simulink model "MaqInd"  (Simulink 8.1)
settings: Solver=ode45  StartTime=0.0  StopTime=1  RelTol=1e-3
InitFcn:
  | clc
  | 
  | %------Simulation parameters-------
  | 
  | Vac = 220/sqrt(3);
  | 
  | Rs = 0.435;
  | Rr = 0.816;
  | Xs = 0.754;
  | Xr = 0.754;
  | Xm = 26.13;
  | 
  | Fe= 60;
  | We = 2*pi*Fe;
  | 
  | Ls = Xs/We;
  | Lr = Xr/We;
  | Lm = Xm/We;
  | 
  | s=0.03;
  | p = 4;
  | Ws=2/p*We;
libraries: powerlib x11
settings Model: Creator=Alves  LastModifiedBy=Alves
settings DataIOCC: SignalLoggingSaveFormat=Dataset
settings OptimizationCC: ExpressionDepthLimit=128
settings DebuggingCC: FcnCallInpInsideContextMsg=EnableAllAsError
settings GRTTargetCC: CombineOutputUpdateFcns=on  GRTInterface=off

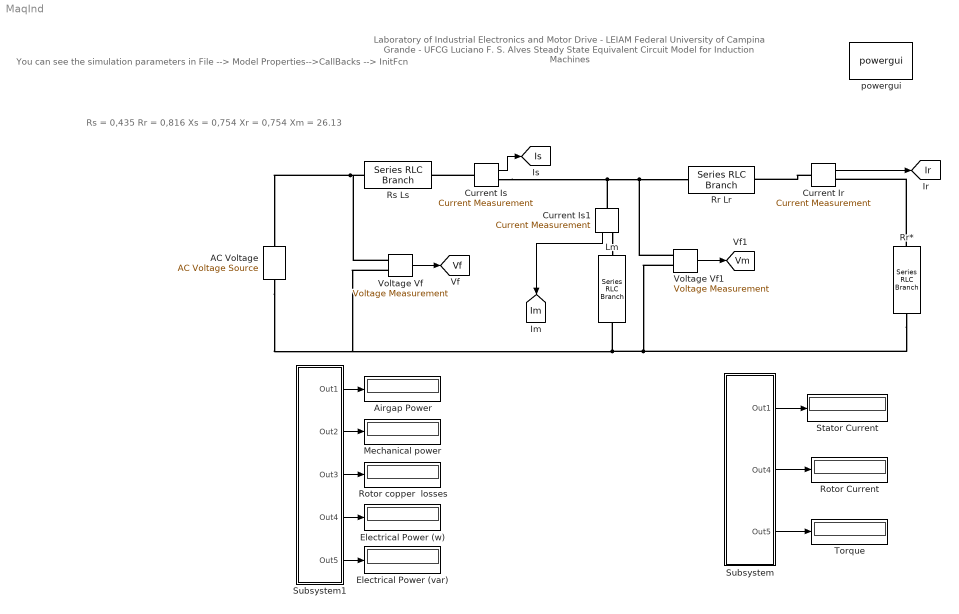
== system MaqInd ==
  note: You can see  the simulation parameters in
      |  File --> Model Properties-->CallBacks --> InitFcn
  note: Rs = 0,435
      | Rr = 0,816
      | Xs = 0,754
      | Xr = 0,754
      | Xm = 26.13
  note: Laboratory of Industrial Electronics and Motor Drive - LEIAM
      | Federal University of Campina Grande - UFCG
      |  Luciano F. S. Alves
      | Steady State Equivalent Circuit Model for Induction Machines
  "AC Voltage " : powerlib/Electrical Sources/AC Voltage Source  Amplitude=Vac  Phase=0  Frequency=Fe  SampleTime=0  Measurements=None
  "Airgap Power " : Display
  Current Ir : powerlib/Measurements/Current Measurement  PhasorSimulation=on  OutputType=Magnitude  PSBequivalent=0
  Current Is : powerlib/Measurements/Current Measurement  PhasorSimulation=on  OutputType=Magnitude  PSBequivalent=0
  Current Is1 : powerlib/Measurements/Current Measurement  PhasorSimulation=on  OutputType=Magnitude  PSBequivalent=0
  Electrical Power (var) : Display
  Electrical Power (w) : Display
  Lm : powerlib/Elements/Series RLC Branch  LConnTagsString=__new0  RConnTagsString=__new0  BranchType=L  Resistance=1  Inductance=Lm  SetiL0=off  InitialCurrent=0  Capacitance=1e-6  Setx0=off  InitialVoltage=0  Measurements=None
  Mechanical power : Display
  "Rotor Current " : Display
  Rotor copper  losses : Display
  Rr Lr : powerlib/Elements/Series RLC Branch  LConnTagsString=__new0  RConnTagsString=__new0  BranchType=RL  Resistance=Rr  Inductance=Lr  SetiL0=off  InitialCurrent=0  Capacitance=1e-6  Setx0=off  InitialVoltage=0  Measurements=None
  Rr* : powerlib/Elements/Series RLC Branch  LConnTagsString=__new0  RConnTagsString=__new0  BranchType=R  Resistance=Rr*((1-s)/s)  Inductance=1e-3  SetiL0=off  InitialCurrent=0  Capacitance=1e-6  Setx0=off  InitialVoltage=0  Measurements=None
  Rs Ls : powerlib/Elements/Series RLC Branch  LConnTagsString=__new0  RConnTagsString=__new0  BranchType=RL  Resistance=Rs  Inductance=Ls  SetiL0=off  InitialCurrent=0  Capacitance=1e-6  Setx0=off  InitialVoltage=0  Measurements=None
  "Stator Current " : Display
  Subsystem : Subsystem
  Subsystem1 : Subsystem
  Torque : Display
  Voltage Vf : powerlib/Measurements/Voltage Measurement  PhasorSimulation=on  OutputType=Magnitude  PSBequivalent=0
  Voltage Vf1 : powerlib/Measurements/Voltage Measurement  PhasorSimulation=on  OutputType=Magnitude  PSBequivalent=0
  powergui : powerlib/powergui  Priority=1  SimulationMode=Phasor  SolverType=Tustin  SampleTime=50e-6  frequency=60  SPID=off  DisableSnubberDevices=off  DisableRonSwitches=off  DisableVfSwitches=off  SwTol=0  Interpol=off  DisplayEquations=off  frequencyindice=60  Pbase=100e6  ErrMax=1e-4  Iterations=50  UnitsV=kV  UnitsW=MW  FunctionMessages=off  echomessages=off  HookPort=off  EnableUseOfTLC=off  x0status=blocks  RestoreLinks=warning  ResistiveCurrentMeasurement=off  Frange=[0:2:500]  Ylog=off  Xlog=on  ShowGrid=off  save=off  variable=ZData  ZoomFFT=off  StartTime=0.0  cycles=1  DisplayStyle=1  fundamental=60  FreqAxis=off  MaxFrequency=1000  frequencyindicesteady=1  RmsSteady=1  display=off  Ts=0  methode=off
  tag scope: Im=global, Ir=global, Is=global, Vf=global, Vm=global
  wires:
  Voltage Vf/1 -> [Vf]
  Current Is/1 -> [Is]
  Current Ir/1 -> [Ir]
  Current Is1/1 -> [Im]
  Voltage Vf1/1 -> [Vm]
  Subsystem/1(Out1) -> "Stator Current "/1
  Subsystem/2(Out4) -> "Rotor Current "/1
  Subsystem/3(Out5) -> Torque/1
  Subsystem1/1(Out1) -> "Airgap Power "/1
  Subsystem1/2(Out2) -> Mechanical power/1
  Subsystem1/3(Out3) -> Rotor copper  losses/1
  Subsystem1/4(Out4) -> Electrical Power (w)/1
  Subsystem1/5(Out5) -> Electrical Power (var)/1
  connections:
  Current Is/RConn1 -- Current Is1/LConn1 -- Voltage Vf1/LConn1 -- Rr Lr/LConn1
  Rr*/RConn1 -- Voltage Vf1/LConn2 -- Voltage Vf/LConn2 -- "AC Voltage "/LConn1 -- Lm/RConn1
  Current Ir/LConn1 -- Rr Lr/RConn1
  Rr*/LConn1 -- Current Ir/RConn1
  Rs Ls/LConn1 -- "AC Voltage "/RConn1 -- Voltage Vf/LConn1
  Current Is/LConn1 -- Rs Ls/RConn1
  Current Is1/RConn1 -- Lm/LConn1

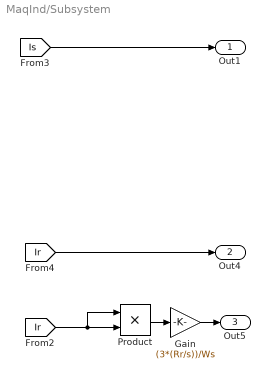
== system MaqInd/Subsystem ==
  Gain : Gain  Gain=(3*(Rr/s))/Ws
  Product : Product
  Out1 : Outport
  Out4 : Outport  Port=2
  Out5 : Outport  Port=3
  wires:
  Gain/1 -> Out5/1
  Product/1 -> Gain/1
  [Ir] -> Out4/1
  [Is] -> Out1/1
  [Ir] -> Product/1, Product/2

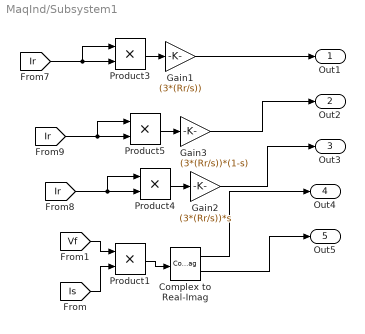
== system MaqInd/Subsystem1 ==
  Complex to Real-Imag : ComplexToRealImag
  Gain1 : Gain  Gain=(3*(Rr/s))
  Gain2 : Gain  Gain=(3*(Rr/s))*s
  Gain3 : Gain  Gain=(3*(Rr/s))*(1-s)
  Product{1,3..5} (4 alike) : Product
  Out1 : Outport
  Out2 : Outport  Port=2
  Out3 : Outport  Port=3
  Out4 : Outport  Port=4
  Out5 : Outport  Port=5
  wires:
  Gain1/1 -> Out1/1
  Gain3/1 -> Out2/1
  Complex to Real-Imag/2 -> Out5/1
  Complex to Real-Imag/1 -> Out4/1
  Gain2/1 -> Out3/1
  Product1/1 -> Complex to Real-Imag/1
  [Is] -> Product1/2
  Product3/1 -> Gain1/1
  [Ir] -> Product3/1, Product3/2
  [Vf] -> Product1/1
  Product5/1 -> Gain3/1
  Product4/1 -> Gain2/1
  [Ir] -> Product4/1, Product4/2
  [Ir] -> Product5/1, Product5/2
